simulink model "ans5"  (R2021a)
settings: Solver=VariableStepAuto  StartTime=0.0  StopTime=1e-3  RelTol=1e-3
undefined symbols (not defined in the file or in its folder): AXI4, Lite, xc7z020clg400
libraries: hdlBasic x47, hlsBasic x2, vmcUtilities x1
settings Model: Creator=cwb21157  LastModifiedBy=abbas
settings SolverCC: AlgebraicLoopSolver=TrustRegion
settings DebuggingCC: SFMachineParentedDataDiag=warning

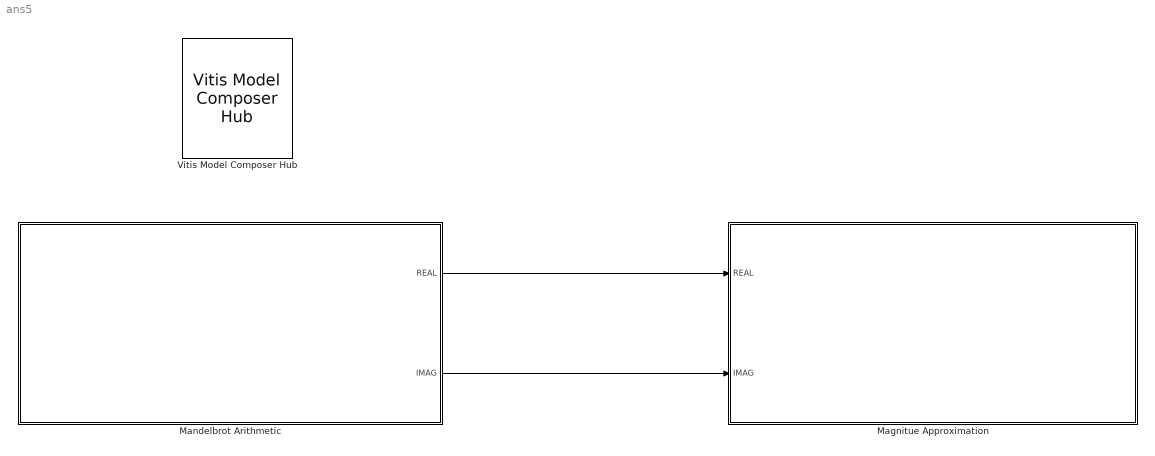
== system ans5 ==
  Magnitue Approximation : Subsystem
  Mandelbrot Arithmetic : Subsystem
  Vitis Model Composer Hub : vmcUtilities/Vitis Model Composer Hub  Tag=genX  CodeGeneration=off  TargetDirectory=./code  ExportType=System Generator  IpVendor=xilinx.com  IpLibrary=hls  IpVersion=1.0  IpHWLanguage=Verilog  AieCompilerOptions={}  AieSimulatorOptions={}  CreateTestbench=off  TestbenchStackSize=10  RunAieSim=off  AieSimTimeout=50000  RunAieSimProfiling=off  LaunchVitisAnalyzer=off  PlotOutput=off  RunX86Sim=off  X86SimTimeout=10  GenHwImage=off  PlatformType=Not Specified  HwSystemType=Baremetal  HwValidationTarget=hw  ProjDevice=xc7z020clg400-1  ProjDevicePart=xc7z020clg400-1  SamplePeriod=-1  ClockFrequency=200  DataPathParallelism=1  xilinxfamily=zynq  part=xc7z020  speed=-1  package=clg400  directory=C:/Users/cwb21157/MANDELBROT  testbench=off  incr_netlist=off  synthesis_tool=Vivado  clock_wrapper=Clock Enables  dbl_ovrd=According to Block Masks  dcm_input_clock_period=10  sysclk_period=10  simulink_period=10e-9  eval_field=0  LogFileName=''  NThreads=4
  wires:
  Mandelbrot Arithmetic/1(REAL) -> Magnitue Approximation/1(REAL)
  Mandelbrot Arithmetic/2(IMAG) -> Magnitue Approximation/2(IMAG)

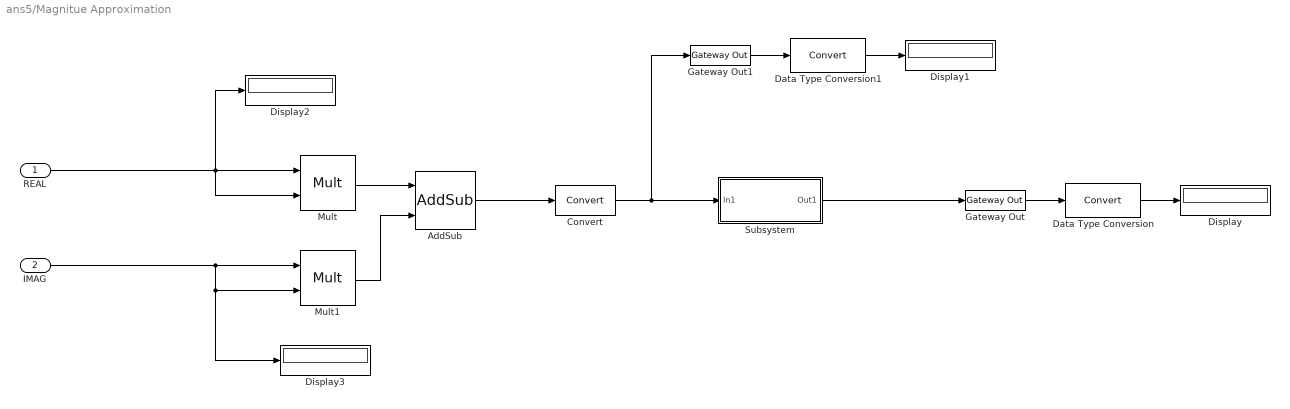
== system ans5/Magnitue Approximation ==
  REAL : Inport
  IMAG : Inport  Port=2
  AddSub : hdlBasic/AddSub  mode=Addition  use_carryin=off  use_carryout=off  en=off  latency=1  precision=User Defined  arith_type=Unsigned  n_bits=20  bin_pt=9  quantization=Truncate  overflow=Wrap  use_behavioral_HDL=off  hw_selection=Fabric  pipelined=on  XmcBlockStatus=1  maskContainerNames=tabcontainer1  block_type=addsub  block_config=sysgen:Addsub_config
  Convert : hdlBasic/Convert  gui_display_data_type=Fixed-point  arith_type=Signed (2's comp)  n_bits=16  bin_pt=6  float_type=Single  exp_bits=8  fraction_bits=24  quantization=Truncate  overflow=Flag as error  en=off  latency=1  pipeline=off  XmcBlockStatus=1  maskContainerNames=group2  block_type=convert  block_config=sysgen:Convert_config  block_width=595  block_height=885
  Data Type Conversion : DataTypeConversion  ConvertRealWorld=Stored Integer (SI)
  Data Type Conversion1 : DataTypeConversion  ConvertRealWorld=Stored Integer (SI)
  Display{,1..3} (4 alike) : Display
      Display settings: Format=decimal (Stored Integer)
      Display2 settings: Format=decimal (Stored Integer)
      Display3 settings: Format=decimal (Stored Integer)
  Gateway Out : hdlBasic/Gateway Out  inherit_from_input=off  hdl_port=on  rows=1  columns=1  UseAsDAC=off  DACChannel='1'  interface=AXI4-Lite  automatic_assignment=on  address_offset=hex2dec('00')  intf_name=''  intf_description=''  timing_constraint=None  locs_specified=off  LOCs={}  io_standard={}  XmcBlockStatus=1  maskContainerNames=group4  block_type=gatewayout  block_config=sysgen:gateway_out_config  block_width_w=590  block_height_w=620  block_width=620  block_height=750
  Gateway Out1 : hdlBasic/Gateway Out  inherit_from_input=off  hdl_port=on  rows=1  columns=1  UseAsDAC=off  DACChannel='1'  interface=AXI4-Lite  automatic_assignment=on  address_offset=hex2dec('00')  intf_name=''  intf_description=''  timing_constraint=None  locs_specified=off  LOCs={}  io_standard={}  XmcBlockStatus=1  maskContainerNames=group4  block_type=gatewayout  block_config=sysgen:gateway_out_config  block_width_w=590  block_height_w=620  block_width=620  block_height=750
  Mult : hdlBasic/Mult  precision=User Defined  arith_type="Signed  (2's comp)"  n_bits=19  bin_pt=6  quantization=Truncate  overflow=Wrap  en=off  latency=3  use_behavioral_HDL=off  opt=Speed  use_embedded=on  optimum_pipeline=off  pipeline=on  use_rpm=on  placement_style=Triangular  XmcBlockStatus=1  maskContainerNames=group1  block_type=mult  block_config=sysgen:Mult_config  block_width=598  block_height=876
  Mult1 : hdlBasic/Mult  precision=User Defined  arith_type="Signed  (2's comp)"  n_bits=19  bin_pt=6  quantization=Truncate  overflow=Wrap  en=off  latency=3  use_behavioral_HDL=off  opt=Speed  use_embedded=on  optimum_pipeline=off  pipeline=on  use_rpm=on  placement_style=Triangular  XmcBlockStatus=1  maskContainerNames=group1  block_type=mult  block_config=sysgen:Mult_config  block_width=598  block_height=876
  Subsystem : Subsystem
  wires:
  Gateway Out/1 -> Data Type Conversion/1
  Data Type Conversion/1 -> Display/1
  REAL/1 -> Display2/1, Mult/2, Mult/1
  IMAG/1 -> Display3/1, Mult1/2, Mult1/1
  Mult/1 -> AddSub/1
  Mult1/1 -> AddSub/2
  AddSub/1 -> Convert/1
  Convert/1 -> Subsystem/1(In1), Gateway Out1/1
  Gateway Out1/1 -> Data Type Conversion1/1
  Data Type Conversion1/1 -> Display1/1
  Subsystem/1(Out1) -> Gateway Out/1

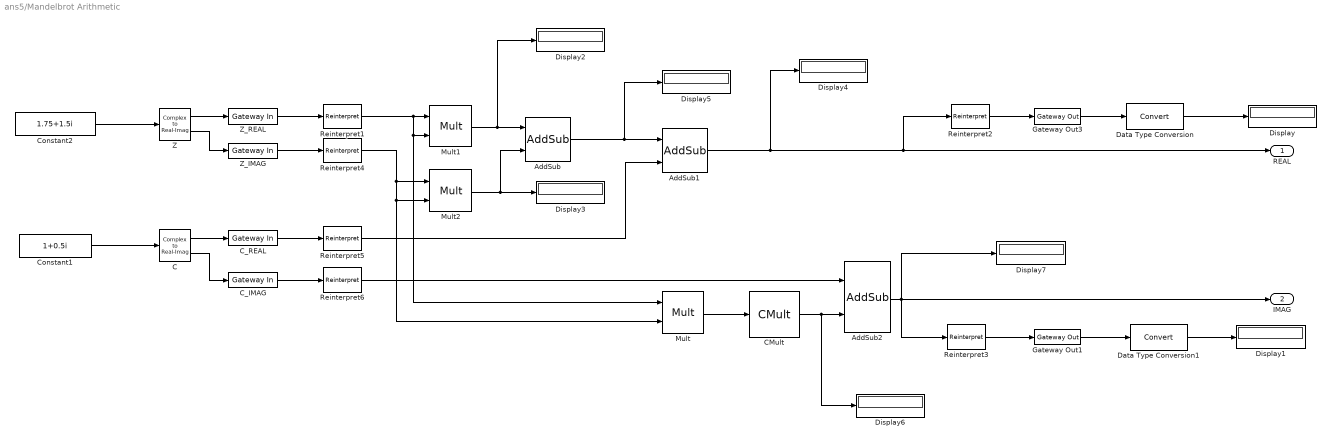
== system ans5/Mandelbrot Arithmetic ==
  AddSub : hdlBasic/AddSub  mode=Subtraction  use_carryin=off  use_carryout=off  en=off  latency=1  precision=User Defined  arith_type="Signed  (2's comp)"  n_bits=16  bin_pt=6  quantization=Truncate  overflow=Wrap  use_behavioral_HDL=off  hw_selection=DSP48  pipelined=on  XmcBlockStatus=1  maskContainerNames=tabcontainer1  block_type=addsub  block_config=sysgen:Addsub_config
  AddSub1 : hdlBasic/AddSub  mode=Addition  use_carryin=off  use_carryout=off  en=off  latency=1  precision=User Defined  arith_type="Signed  (2's comp)"  n_bits=32  bin_pt=6  quantization=Truncate  overflow=Wrap  use_behavioral_HDL=off  hw_selection=DSP48  pipelined=on  XmcBlockStatus=1  maskContainerNames=tabcontainer1  block_type=addsub  block_config=sysgen:Addsub_config
  AddSub2 : hdlBasic/AddSub  mode=Addition  use_carryin=off  use_carryout=off  en=off  latency=1  precision=User Defined  arith_type="Signed  (2's comp)"  n_bits=19  bin_pt=6  quantization=Truncate  overflow=Wrap  use_behavioral_HDL=off  hw_selection=DSP48  pipelined=on  XmcBlockStatus=1  maskContainerNames=tabcontainer1  block_type=addsub  block_config=sysgen:Addsub_config
  C : hlsBasic/Complex to Real-Imag  Output=Real and imag
  CMult : hdlBasic/CMult  const=2  gui_display_data_type=Fixed-point  const_n_bits=18  const_bin_pt=6  float_type=Single  exp_bits=8  fraction_bits=24  en=off  latency=1  precision=User Defined  arith_type="Signed  (2's comp)"  n_bits=32  bin_pt=9  quantization=Truncate  overflow=Wrap  use_behavioral_HDL=off  mem_type=Block RAM  pipeline=off  XmcBlockStatus=1  maskContainerNames=tabcontainer1  block_type=cmult  block_config=sysgen:CMult_config
      settings: infoedit=[]
  C_IMAG : hdlBasic/Gateway In  gui_display_data_type=Fixed-point  arith_type=Signed (2's comp)  n_bits=16  bin_pt=3  preci_type=Single  exp_width=8  frac_width=24  rows=1  columns=1  quantization="Round  (unbiased: +/- Inf)"  overflow=Saturate  period=10e-9  UseAsADC=off  ADCChannel='1'  interface=AXI4-Lite  automatic_assignment=on  address_offset=hex2dec('00')  intf_name=''  intf_description=''  default_value=0  timing_constraint=None  locs_specified=off  LOCs={}  io_standard={}  inherit_from_input=off  hdl_port=on  XmcBlockStatus=1  maskContainerNames=group4  block_type=gatewayin  block_config=sysgen:gateway_in_config  block_width_w=590  block_height_w=620  block_width=640  block_height=850
  C_REAL : hdlBasic/Gateway In  gui_display_data_type=Fixed-point  arith_type=Signed (2's comp)  n_bits=16  bin_pt=3  preci_type=Single  exp_width=8  frac_width=24  rows=1  columns=1  quantization="Round  (unbiased: +/- Inf)"  overflow=Saturate  period=10e-9  UseAsADC=off  ADCChannel='1'  interface=AXI4-Lite  automatic_assignment=on  address_offset=hex2dec('00')  intf_name=''  intf_description=''  default_value=0  timing_constraint=None  locs_specified=off  LOCs={}  io_standard={}  inherit_from_input=off  hdl_port=on  XmcBlockStatus=1  maskContainerNames=group4  block_type=gatewayin  block_config=sysgen:gateway_in_config  block_width_w=590  block_height_w=620  block_width=640  block_height=850
  Constant1 : Constant  Value=1+0.5i  SampleTime=10e-9
  Constant2 : Constant  Value=1.75+1.5i  SampleTime=10e-9
  Data Type Conversion : DataTypeConversion  ConvertRealWorld=Stored Integer (SI)
  Data Type Conversion1 : DataTypeConversion  ConvertRealWorld=Stored Integer (SI)
  Display{,1..7} (8 alike) : Display
      settings: Format=decimal (Stored Integer)
  Gateway Out1 : hdlBasic/Gateway Out  inherit_from_input=off  hdl_port=on  rows=1  columns=1  UseAsDAC=off  DACChannel='1'  interface=AXI4-Lite  automatic_assignment=on  address_offset=hex2dec('00')  intf_name=''  intf_description=''  timing_constraint=None  locs_specified=off  LOCs={}  io_standard={}  XmcBlockStatus=1  maskContainerNames=group4  block_type=gatewayout  block_config=sysgen:gateway_out_config  block_width_w=590  block_height_w=620  block_width=620  block_height=750
  Gateway Out3 : hdlBasic/Gateway Out  inherit_from_input=off  hdl_port=on  rows=1  columns=1  UseAsDAC=off  DACChannel='1'  interface=AXI4-Lite  automatic_assignment=on  address_offset=hex2dec('00')  intf_name=''  intf_description=''  timing_constraint=None  locs_specified=off  LOCs={}  io_standard={}  XmcBlockStatus=1  maskContainerNames=group4  block_type=gatewayout  block_config=sysgen:gateway_out_config  block_width_w=590  block_height_w=620  block_width=620  block_height=750
  Mult : hdlBasic/Mult  precision=User Defined  arith_type="Signed  (2's comp)"  n_bits=16  bin_pt=6  quantization=Truncate  overflow=Wrap  en=off  latency=3  use_behavioral_HDL=off  opt=Speed  use_embedded=on  optimum_pipeline=on  pipeline=on  use_rpm=on  placement_style=Triangular  XmcBlockStatus=1  maskContainerNames=group1  block_type=mult  block_config=sysgen:Mult_config  block_width=598  block_height=876
  Mult1 : hdlBasic/Mult  precision=User Defined  arith_type="Signed  (2's comp)"  n_bits=16  bin_pt=6  quantization=Truncate  overflow=Wrap  en=off  latency=3  use_behavioral_HDL=off  opt=Speed  use_embedded=on  optimum_pipeline=on  pipeline=on  use_rpm=on  placement_style=Triangular  XmcBlockStatus=1  maskContainerNames=group1  block_type=mult  block_config=sysgen:Mult_config  block_width=598  block_height=876
  Mult2 : hdlBasic/Mult  precision=User Defined  arith_type="Signed  (2's comp)"  n_bits=16  bin_pt=6  quantization=Truncate  overflow=Wrap  en=off  latency=3  use_behavioral_HDL=off  opt=Speed  use_embedded=on  optimum_pipeline=on  pipeline=on  use_rpm=on  placement_style=Triangular  XmcBlockStatus=1  maskContainerNames=group1  block_type=mult  block_config=sysgen:Mult_config  block_width=598  block_height=876
  Reinterpret{1,4..6} (4 alike) : hdlBasic/Reinterpret  force_arith_type=off  arith_type=Unsigned  force_bin_pt=on  bin_pt=3  XmcBlockStatus=1  maskContainerNames=group1  block_type=reinterpret  block_config=sysgen:Reinterpret_config
  Reinterpret2 : hdlBasic/Reinterpret  force_arith_type=on  arith_type=Unsigned  force_bin_pt=off  bin_pt=0  XmcBlockStatus=1  maskContainerNames=group1  block_type=reinterpret  block_config=sysgen:Reinterpret_config
  Reinterpret3 : hdlBasic/Reinterpret  force_arith_type=on  arith_type=Unsigned  force_bin_pt=off  bin_pt=0  XmcBlockStatus=1  maskContainerNames=group1  block_type=reinterpret  block_config=sysgen:Reinterpret_config
  Z : hlsBasic/Complex to Real-Imag  Output=Real and imag
  Z_IMAG : hdlBasic/Gateway In  gui_display_data_type=Fixed-point  arith_type=Signed (2's comp)  n_bits=16  bin_pt=3  preci_type=Single  exp_width=8  frac_width=24  rows=1  columns=1  quantization="Round  (unbiased: +/- Inf)"  overflow=Saturate  period=10e-9  UseAsADC=off  ADCChannel='1'  interface=AXI4-Lite  automatic_assignment=on  address_offset=hex2dec('00')  intf_name=''  intf_description=''  default_value=0  timing_constraint=None  locs_specified=off  LOCs={}  io_standard={}  inherit_from_input=off  hdl_port=on  XmcBlockStatus=1  maskContainerNames=group4  block_type=gatewayin  block_config=sysgen:gateway_in_config  block_width_w=590  block_height_w=620  block_width=640  block_height=850
  Z_REAL : hdlBasic/Gateway In  gui_display_data_type=Fixed-point  arith_type=Signed (2's comp)  n_bits=16  bin_pt=3  preci_type=Single  exp_width=8  frac_width=24  rows=1  columns=1  quantization="Round  (unbiased: +/- Inf)"  overflow=Saturate  period=10e-9  UseAsADC=off  ADCChannel='1'  interface=AXI4-Lite  automatic_assignment=on  address_offset=hex2dec('00')  intf_name=''  intf_description=''  default_value=0  timing_constraint=None  locs_specified=off  LOCs={}  io_standard={}  inherit_from_input=off  hdl_port=on  XmcBlockStatus=1  maskContainerNames=group4  block_type=gatewayin  block_config=sysgen:gateway_in_config  block_width_w=590  block_height_w=620  block_width=640  block_height=850
  REAL : Outport
  IMAG : Outport  Port=2
  wires:
  Z_IMAG/1 -> Reinterpret4/1
  Mult1/1 -> Display2/1, AddSub/1
  Mult2/1 -> Display3/1, AddSub/2
  AddSub/1 -> Display5/1, AddSub1/1
  C_REAL/1 -> Reinterpret5/1
  AddSub1/1 -> Display4/1, REAL/1, Reinterpret2/1
  Mult/1 -> CMult/1
  C_IMAG/1 -> Reinterpret6/1
  AddSub2/1 -> Display7/1, Reinterpret3/1, IMAG/1
  Data Type Conversion/1 -> Display/1
  Reinterpret2/1 -> Gateway Out3/1
  Reinterpret3/1 -> Gateway Out1/1
  Z_REAL/1 -> Reinterpret1/1
  Reinterpret1/1 -> Mult1/2, Mult/1, Mult1/1
  Constant2/1 -> Z/1
  Constant1/1 -> C/1
  Reinterpret4/1 -> Mult/2, Mult2/2, Mult2/1
  Reinterpret5/1 -> AddSub1/2
  Data Type Conversion1/1 -> Display1/1
  Gateway Out3/1 -> Data Type Conversion/1
  Gateway Out1/1 -> Data Type Conversion1/1
  CMult/1 -> Display6/1, AddSub2/2
  Reinterpret6/1 -> AddSub2/1
  C/1 -> C_REAL/1
  C/2 -> C_IMAG/1
  Z/1 -> Z_REAL/1
  Z/2 -> Z_IMAG/1

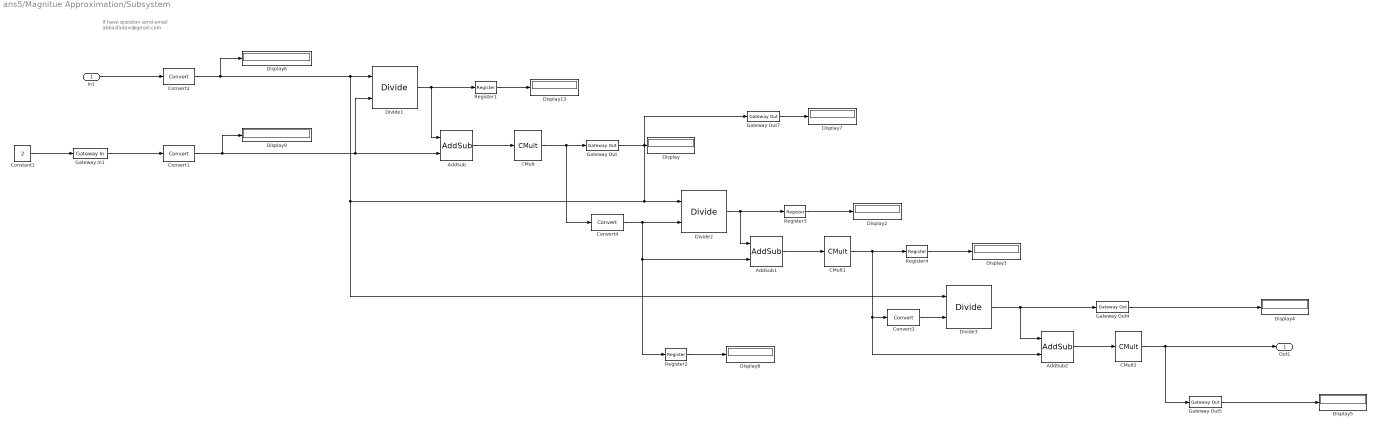
== system ans5/Magnitue Approximation/Subsystem ==
  note: if have question send email
      | abbasfadavi@gmail.com
  In1 : Inport
  AddSub : hdlBasic/AddSub  mode=Addition  use_carryin=off  use_carryout=off  en=off  latency=0  precision=Full  arith_type="Signed  (2's comp)"  n_bits=20  bin_pt=8  quantization=Truncate  overflow=Wrap  use_behavioral_HDL=off  hw_selection=DSP48  pipelined=off  XmcBlockStatus=1  maskContainerNames=tabcontainer1  block_type=addsub  block_config=sysgen:Addsub_config
  AddSub1 : hdlBasic/AddSub  mode=Addition  use_carryin=off  use_carryout=off  en=off  latency=0  precision=Full  arith_type="Signed  (2's comp)"  n_bits=20  bin_pt=8  quantization=Truncate  overflow=Wrap  use_behavioral_HDL=off  hw_selection=DSP48  pipelined=off  XmcBlockStatus=1  maskContainerNames=tabcontainer1  block_type=addsub  block_config=sysgen:Addsub_config
  AddSub2 : hdlBasic/AddSub  mode=Addition  use_carryin=off  use_carryout=off  en=off  latency=0  precision=Full  arith_type="Signed  (2's comp)"  n_bits=20  bin_pt=8  quantization=Truncate  overflow=Wrap  use_behavioral_HDL=off  hw_selection=DSP48  pipelined=off  XmcBlockStatus=1  maskContainerNames=tabcontainer1  block_type=addsub  block_config=sysgen:Addsub_config
  CMult : hdlBasic/CMult  const=0.5  gui_display_data_type=Fixed-point  const_n_bits=10  const_bin_pt=8  float_type=Single  exp_bits=8  fraction_bits=8  en=off  latency=0  precision=Full  arith_type="Signed  (2's comp)"  n_bits=16  bin_pt=14  quantization=Truncate  overflow=Wrap  use_behavioral_HDL=off  mem_type=Distributed RAM  pipeline=off  XmcBlockStatus=1  maskContainerNames=tabcontainer1  block_type=cmult  block_config=sysgen:CMult_config
      settings: infoedit=[]
  CMult1 : hdlBasic/CMult  const=0.5  gui_display_data_type=Fixed-point  const_n_bits=10  const_bin_pt=8  float_type=Single  exp_bits=8  fraction_bits=8  en=off  latency=0  precision=Full  arith_type="Signed  (2's comp)"  n_bits=16  bin_pt=14  quantization=Truncate  overflow=Wrap  use_behavioral_HDL=off  mem_type=Distributed RAM  pipeline=off  XmcBlockStatus=1  maskContainerNames=tabcontainer1  block_type=cmult  block_config=sysgen:CMult_config
      settings: infoedit=[]
  CMult2 : hdlBasic/CMult  const=0.5  gui_display_data_type=Fixed-point  const_n_bits=10  const_bin_pt=8  float_type=Single  exp_bits=8  fraction_bits=8  en=off  latency=0  precision=Full  arith_type="Signed  (2's comp)"  n_bits=16  bin_pt=14  quantization=Truncate  overflow=Wrap  use_behavioral_HDL=off  mem_type=Distributed RAM  pipeline=off  XmcBlockStatus=1  maskContainerNames=tabcontainer1  block_type=cmult  block_config=sysgen:CMult_config
      settings: infoedit=[]
  Constant1 : Constant  Value=2
  Convert{1..4} (4 alike) : hdlBasic/Convert  gui_display_data_type=Fixed-point  arith_type=Signed (2's comp)  n_bits=16  bin_pt=4  float_type=Single  exp_bits=8  fraction_bits=8  quantization=Truncate  overflow=Wrap  en=off  latency=0  pipeline=off  XmcBlockStatus=1  maskContainerNames=group2  block_type=convert  block_config=sysgen:Convert_config  block_width=595  block_height=885
  Display{,2..9,13} (10 alike) : Display
      settings: Format=decimal (Stored Integer)
  Divide1 : hdlBasic/Divide  flow_control=NonBlocking  axi_optimize_goal=Resources  algorithm_type=Radix2  fractional_width=8  latency=0  rate=1  has_a_tlast=off  has_a_tuser=off  has_b_tlast=off  has_b_tuser=off  en=off  has_result_tready=off  result_tlast_behv=Pass_A_TLAST  has_underflow=off  has_overflow=off  has_invalid_op=off  has_divide_by_zero=off  fpo_op_type=mergeddivide  XmcBlockStatus=1  maskContainerNames=tabcontainer1  block_type=divide  block_config=sysgen:FPOBlockDescriptor_config
  Divide2 : hdlBasic/Divide  flow_control=NonBlocking  axi_optimize_goal=Resources  algorithm_type=Radix2  fractional_width=8  latency=0  rate=1  has_a_tlast=off  has_a_tuser=off  has_b_tlast=off  has_b_tuser=off  en=off  has_result_tready=off  result_tlast_behv=Pass_A_TLAST  has_underflow=off  has_overflow=off  has_invalid_op=off  has_divide_by_zero=off  fpo_op_type=mergeddivide  XmcBlockStatus=1  maskContainerNames=tabcontainer1  block_type=divide  block_config=sysgen:FPOBlockDescriptor_config
  Divide3 : hdlBasic/Divide  flow_control=NonBlocking  axi_optimize_goal=Resources  algorithm_type=Radix2  fractional_width=8  latency=0  rate=1  has_a_tlast=off  has_a_tuser=off  has_b_tlast=off  has_b_tuser=off  en=off  has_result_tready=off  result_tlast_behv=Pass_A_TLAST  has_underflow=off  has_overflow=off  has_invalid_op=off  has_divide_by_zero=off  fpo_op_type=mergeddivide  XmcBlockStatus=1  maskContainerNames=tabcontainer1  block_type=divide  block_config=sysgen:FPOBlockDescriptor_config
  Gateway In1 : hdlBasic/Gateway In  gui_display_data_type=Fixed-point  arith_type=Signed (2's comp)  n_bits=16  bin_pt=6  preci_type=Single  exp_width=8  frac_width=24  rows=1  columns=1  quantization="Round  (unbiased: +/- Inf)"  overflow=Saturate  period=10e-9  UseAsADC=off  ADCChannel='1'  interface=AXI4-Lite  automatic_assignment=on  address_offset=hex2dec('00')  intf_name=''  intf_description=''  default_value=0  timing_constraint=None  locs_specified=off  LOCs={}  io_standard={}  inherit_from_input=off  hdl_port=on  XmcBlockStatus=1  maskContainerNames=group4  block_type=gatewayin  block_config=sysgen:gateway_in_config  block_width_w=590  block_height_w=620  block_width=640  block_height=850
  Gateway Out{,4..5,7} (4 alike) : hdlBasic/Gateway Out  inherit_from_input=off  hdl_port=on  rows=1  columns=1  UseAsDAC=off  DACChannel='1'  interface=AXI4-Lite  automatic_assignment=on  address_offset=hex2dec('00')  intf_name=''  intf_description=''  timing_constraint=None  locs_specified=off  LOCs={}  io_standard={}  XmcBlockStatus=1  maskContainerNames=group4  block_type=gatewayout  block_config=sysgen:gateway_out_config  block_width_w=590  block_height_w=620  block_width=620  block_height=750
  Register{1..4} (4 alike) : hdlBasic/Register  init=0  rst=off  en=off  XmcBlockStatus=1  maskContainerNames=tabcontainer1  block_type=register  block_config=sysgen:Register_config
  Out1 : Outport
  wires:
  AddSub1/1 -> CMult1/1
  Divide2/1 -> Register3/1, AddSub1/1
  Gateway Out5/1 -> Display5/1
  Gateway Out4/1 -> Display4/1
  Gateway In1/1 -> Convert1/1
  Constant1/1 -> Gateway In1/1
  CMult1/1 -> Register4/1, AddSub2/2, Convert3/1
  In1/1 -> Convert2/1
  AddSub2/1 -> CMult2/1
  Divide3/1 -> Gateway Out4/1, AddSub2/1
  Gateway Out/1 -> Display/1
  AddSub/1 -> CMult/1
  CMult2/1 -> Out1/1, Gateway Out5/1
  Divide1/1 -> Register1/1, AddSub/1
  Gateway Out7/1 -> Display7/1
  CMult/1 -> Convert4/1, Gateway Out/1
  Register2/1 -> Display8/1
  Convert1/1 -> Divide1/2, AddSub/2, Display9/1
  Register1/1 -> Display13/1
  Convert2/1 -> Display6/1, Divide1/1, Gateway Out7/1, Divide2/1, Divide3/1
  Convert4/1 -> AddSub1/2, Register2/1, Divide2/2
  Register3/1 -> Display2/1
  Register4/1 -> Display3/1
  Convert3/1 -> Divide3/2
